simulink model "Ejer10TemperaturaSobreSuelo"  (R2023b)
settings: Solver=FixedStepAuto  StartTime=0  StopTime=499  FixedStep=1  RelTol=1e-3
settings Model: Creator=alfre  LastModifiedBy=alfre

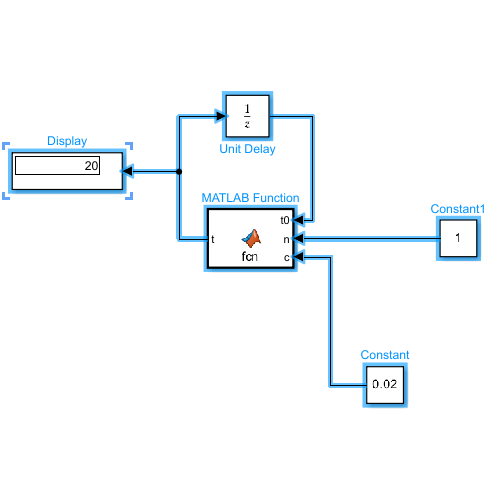
[thumbnail: Simulink's stored preview of the top-level diagram]
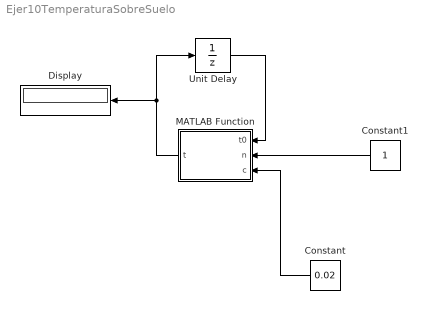
== system Ejer10TemperaturaSobreSuelo ==
  Constant : Constant  Value=0.02
  Constant1 : Constant
  Display : Display
  MATLAB Function : MATLAB Function  TreatAsAtomicUnit=on
  Unit Delay : UnitDelay  InitialCondition=30  SampleTime=-1  HasFrameUpgradeWarning=on
  wires:
  Unit Delay/1 -> MATLAB Function/1(t0)
  MATLAB Function/1(t) -> Display/1, Unit Delay/1
  Constant/1 -> MATLAB Function/3(c)
  Constant1/1 -> MATLAB Function/2(n)

== matlab function Ejer10TemperaturaSobreSuelo/MATLAB Function ==
  data: t0 input; t output; n input; c input
function t = fcn(t0, n, c)

t = t0 - n*c;
